simulink model "Model"  (R2023a)
settings: Solver=ode23s  StartTime=0.0  StopTime=60  RelTol=1e-3
values from neighbouring files (symbols this model uses):
  Num_of_Signals = h    [DataSet_generator.m]
  X0 = [0;0;0]    [DataSet_generator.m]
settings Model: Creator=sepeh  LastModifiedBy=sepeh

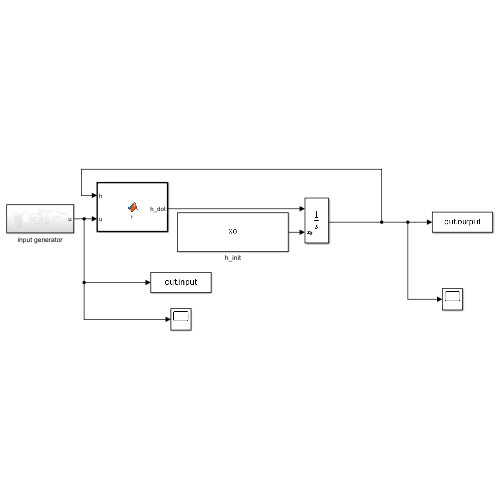
[thumbnail: Simulink's stored preview of the top-level diagram]
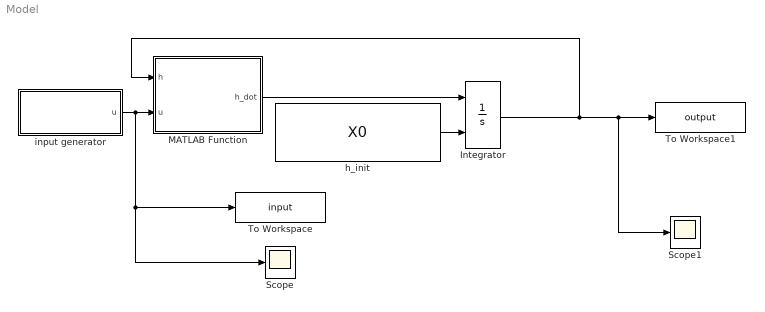
== system Model ==
  Integrator : Integrator  InitialConditionSource=external
  MATLAB Function : MATLAB Function  TreatAsAtomicUnit=on
  Scope : Scope
  Scope1 : Scope
  To Workspace : ToWorkspace  VariableName=input  SaveFormat=Timeseries  SampleTime=0.01
  To Workspace1 : ToWorkspace  VariableName=output  SaveFormat=Timeseries  SampleTime=0.01
  h_init : Constant  Value=X0
  input generator : Subsystem
  wires:
  h_init/1 -> Integrator/2
  MATLAB Function/1(h_dot) -> Integrator/1
  Integrator/1 -> Scope1/1, To Workspace1/1, MATLAB Function/1(h)
  input generator/1(u) -> Scope/1, To Workspace/1, MATLAB Function/2(u)

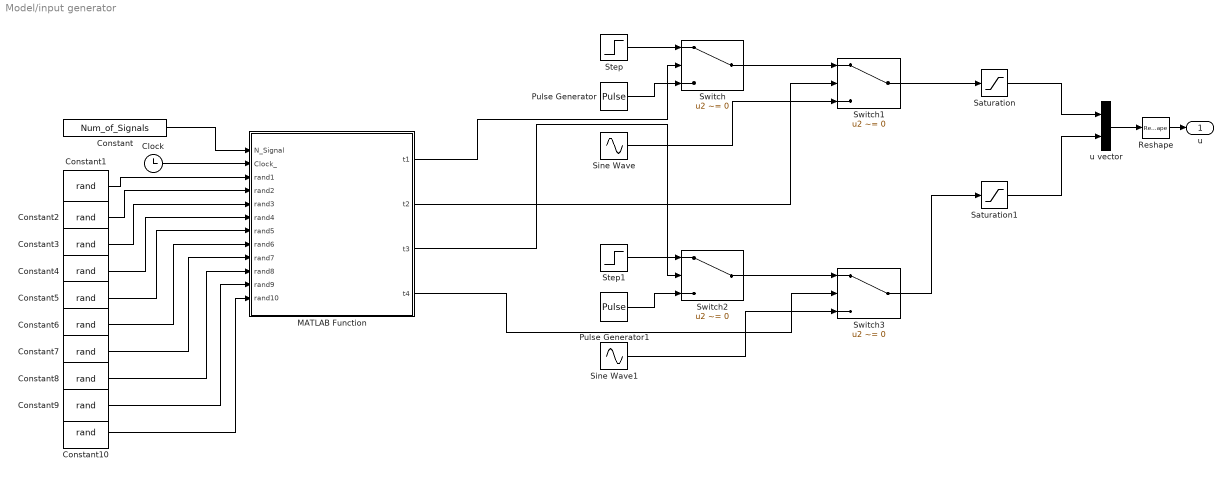
== system Model/input generator ==
  Clock : Clock
  Constant : Constant  Value=Num_of_Signals
  Constant{1..10} (10 alike) : Constant  Value=rand
  MATLAB Function : MATLAB Function  TreatAsAtomicUnit=on
  Pulse Generator : DiscretePulseGenerator  PulseType=Time based  Amplitude=rand*250  Period=rand*60  PulseWidth=rand*100
  Pulse Generator1 : DiscretePulseGenerator  PulseType=Time based  Amplitude=rand*250  Period=rand*60  PulseWidth=rand*100
  Reshape : Reshape  OutputDimensionality=Column vector (2-D)
  Saturation : Saturate  UpperLimit=250  LowerLimit=0
  Saturation1 : Saturate  UpperLimit=250  LowerLimit=0
  Sine Wave : Sin  Amplitude=rand*125  Bias=125  Frequency=((pi)-1.053e-01)*rand + 1.053e-01  SampleTime=0
  Sine Wave1 : Sin  Amplitude=rand*125  Bias=125  Frequency=((pi)-1.053e-01)*rand + 1.053e-01  SampleTime=0
  Step : Step  Time=rand*60  After=rand*250  SampleTime=0
  Step1 : Step  Time=rand*60  After=rand*250  SampleTime=0
  Switch{,1..3} (4 alike) : Switch  Criteria=u2 ~= 0  Threshold=rand*300  SaturateOnIntegerOverflow=off  InputSameDT=off
  u vector : Concatenate
  u : Outport
  wires:
  u vector/1 -> Reshape/1
  Reshape/1 -> u/1
  Saturation/1 -> u vector/1
  Saturation1/1 -> u vector/2
  Pulse Generator/1 -> Switch/3
  Switch2/1 -> Switch3/1
  Switch/1 -> Switch1/1
  Pulse Generator1/1 -> Switch2/3
  Step/1 -> Switch/1
  Step1/1 -> Switch2/1
  Switch3/1 -> Saturation1/1
  Switch1/1 -> Saturation/1
  Sine Wave1/1 -> Switch3/3
  Sine Wave/1 -> Switch1/3
  MATLAB Function/1(t1) -> Switch/2
  MATLAB Function/2(t2) -> Switch1/2
  MATLAB Function/3(t3) -> Switch2/2
  MATLAB Function/4(t4) -> Switch3/2
  Clock/1 -> MATLAB Function/2(Clock_)
  Constant/1 -> MATLAB Function/1(N_Signal)
  Constant1/1 -> MATLAB Function/3(rand1)
  Constant2/1 -> MATLAB Function/4(rand2)
  Constant3/1 -> MATLAB Function/5(rand3)
  Constant4/1 -> MATLAB Function/6(rand4)
  Constant5/1 -> MATLAB Function/7(rand5)
  Constant6/1 -> MATLAB Function/8(rand6)
  Constant7/1 -> MATLAB Function/9(rand7)
  Constant8/1 -> MATLAB Function/10(rand8)
  Constant9/1 -> MATLAB Function/11(rand9)
  Constant10/1 -> MATLAB Function/12(rand10)

== matlab function Model/input generator/MATLAB Function ==
  data: t1 output; t2 output; t3 output; t4 output; N_Signal input; Clock_ input; rand1 input; rand2 input; rand3 input; rand4 input; rand5 input; rand6 input; rand7 input; rand8 input; rand9 input; rand10 input
function [t1,t2,t3,t4]= time_manager(N_Signal,Clock_,rand1,rand2,rand3,rand4,rand5,rand6,rand7,rand8,rand9,rand10)
t1=0;
t2=0;
t3=0;
t4=0;
period=60;
if N_Signal<=1
    [t1,t2]=Switch_selector(rand1*3);
    [t3,t4]=Switch_selector(rand2*3);
elseif N_Signal<=2
    change_time1=rand1*period;
    if(change_time1>=Clock_)
        [t1,t2]=Switch_selector(rand2*3);
    else
        [t1,t2]=Switch_selector(rand3*3);
    end
    change_time2=rand2*period;
    if(change_time2>=Clock_)
        [t3,t4]=Switch_selector(rand4*3);
    else
        [t3,t4]=Switch_selector(rand5*3);
    end
else
    change_time_1_1=rand1*period;
    change_time_1_2=(period-change_time_1_1)*rand2+change_time_1_1;
    change_time_2_1=rand3*period;
    change_time_2_2=(period-change_time_2_1)*rand4+change_time_2_1;
    if change_time_1_1>Clock_
        [t1,t2]=Switch_selector(rand5*3);
    elseif change_time_1_1<=Clock_ && change_time_1_2>=Clock_
        [t1,t2]=Switch_selector(rand6*3);
    elseif change_time_1_2<Clock_
        [t1,t2]=Switch_selector(rand7*3);
    end
    if change_time_2_1>Clock_
        [t3,t4]=Switch_selector(rand8*3);
    elseif change_time_2_1<=Clock_ && change_time_2_2>=Clock_
        [t3,t4]=Switch_selector(rand9*3);
    elseif change_time_2_2<Clock_
        [t3,t4]=Switch_selector(rand10*3);
    end
end

== matlab function Model/MATLAB Function ==
  data: h input; u input; h_dot output
function h_dot = f(h,u)
g=1000;
A=154;
a1=0.46;
a2=0.6;
a3=0.45;
S13=0.5;
S23=0.5;
S2o=0.5;
Q13=a1*S13*sign(h(1)-h(3))*sqrt(2*g*abs(h(1)-h(3)));
Q23=a3*S23*sign(h(3)-h(2))*sqrt(2*g*abs(h(3)-h(2)));
Q2o=a2*S2o*sqrt(abs(2*g*h(2)));
h_dot = 1/A*[u(1)-Q13;u(2)+Q23-Q2o;Q13-Q23];
